simulink model "gm_filter_low_pass_simulink"  (R2025a)
settings: Solver=FixedStepAuto  StartTime=0.0  StopTime=10e-3  MaxStep=1/(44e3)  RelTol=1e-3  EnableMultiTasking=on
settings Model: Creator=thiag  LastModifiedBy=thiag
settings SolverCC: PositivePriorityOrder=on
settings OptimizationCC: BlockReduction=off  ConditionallyExecuteInputs=off  DefaultParameterBehavior=Inlined  UseDivisionForNetSlopeComputation=on  GainParamInheritBuiltInType=on  DefaultUnderspecifiedDataType=single  EnhancedBackFolding=on  PassReuseOutputArgsAs=Individual arguments  ZeroExternalMemoryAtStartup=off  ZeroInternalMemoryAtStartup=off  MaxStackSize=64  OptimizeBlockOrder=speed  DifferentSizesBufferReuse=on  OptimizationCustomize=off  EfficientTunableParamExpr=on
settings DebuggingCC: InheritedTsInSrcMsg=none  ParameterTunabilityLossMsg=error
settings HardwareCC: ProdBitPerPointer=32.0  ProdBitPerSizeT=32.0  ProdBitPerPtrDiffT=32.0  ProdLargestAtomicInteger=Long  ProdLargestAtomicFloat=Double  ProdWordSize=32.0  ProdLongLongMode=on  ProdHWDeviceType=ARM Compatible->ARM Cortex-A (32-bit)
settings SFSimCC: MATLABDynamicMemAlloc=off
settings RTWCC: SystemTargetFile=ert.tlc  HardwareBoard=Arrow SoCKit development board  TLCOptions="-aInlineSetEventsForThisBaseRateFcn=TLC_FALSE -aSuppressMultiTaskScheduler=TLC_FALSE  -aRateBasedStepFcn=0"  TemplateMakefile=ert_default_tmf  GenerateReport=on  Toolchain=ARM Development Studio Altera Edition (DS-5 AE)  LaunchReport=on  GenerateWebview=on  Description=Embedded Coder
settings CodeAppCC: ForceParamTrailComments=on  IgnoreCustomStorageClasses=off  OperatorAnnotations=on  SimulinkDataObjDesc=on  SFDataObjDesc=on  InsertBlockDesc=on
settings ERTTargetCC: ExtModeTransport=0.0  ExtModeStaticAlloc=off  ExtModeMexFile=ext_comm  ExtModeIntrfLevel=Level1

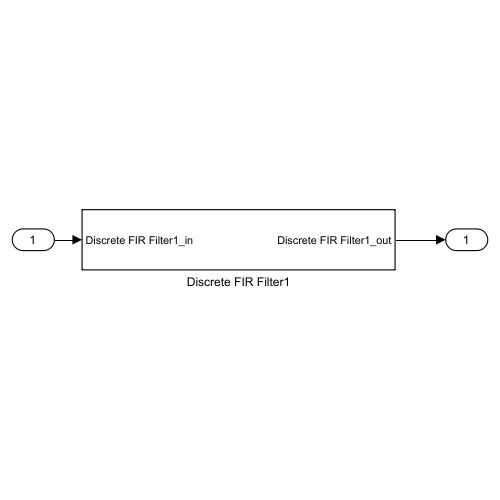
[thumbnail: Simulink's stored preview of the top-level diagram]
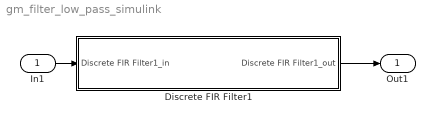
== system gm_filter_low_pass_simulink ==
  In1 : Inport  OutDataTypeStr=single  PortDimensions=1  SampleTime=0.0002
  Discrete FIR Filter1 : Subsystem
  Out1 : Outport  SampleTime=0.0002  VectorParamsAs1DForOutWhenUnconnected=off
  wires:
  In1/1 -> Discrete FIR Filter1/1(Discrete FIR Filter1_in)
  Discrete FIR Filter1/1(Discrete FIR Filter1_out) -> Out1/1

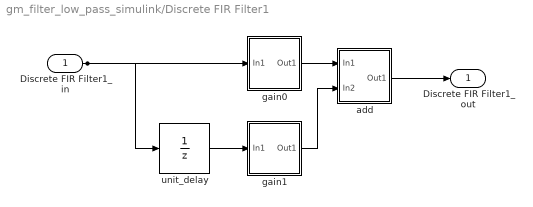
== system gm_filter_low_pass_simulink/Discrete FIR Filter1 ==
  Discrete FIR Filter1_in : Inport  OutDataTypeStr=single  SampleTime=0.0002
  add : Subsystem
      mask Display: disp('NFP\nadd');
  gain0 : Subsystem
      mask Display: disp('NFP\ngain_pow2');
  gain1 : Subsystem
      mask Display: disp('NFP\ngain_pow2');
  unit_delay : UnitDelay  InitialCondition=double(0)  SampleTime=0.0002
  Discrete FIR Filter1_out : Outport  OutDataTypeStr=single  SampleTime=0.0002
  wires:
  Discrete FIR Filter1_in/1 -> gain0/1(In1), unit_delay/1
  unit_delay/1 -> gain1/1(In1)
  gain0/1(Out1) -> add/1(In1)
  add/1(Out1) -> Discrete FIR Filter1_out/1
  gain1/1(Out1) -> add/2(In2)

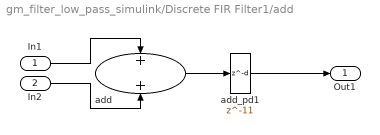
== system gm_filter_low_pass_simulink/Discrete FIR Filter1/add ==
  In1 : Inport
  In2 : Inport  Port=2
  add : Sum  OutDataTypeStr=single  SampleTime=0.0002
  add_pd1 : Delay  DelayLength=11
  Out1 : Outport
  wires:
  In1/1 -> add/1
  In2/1 -> add/2
  add/1 -> add_pd1/1
  add_pd1/1 -> Out1/1

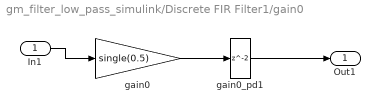
== system gm_filter_low_pass_simulink/Discrete FIR Filter1/gain0 ==
  In1 : Inport
  gain0 : Gain  Gain=single(0.5)
  gain0_pd1 : Delay
  Out1 : Outport
  wires:
  In1/1 -> gain0/1
  gain0/1 -> gain0_pd1/1
  gain0_pd1/1 -> Out1/1

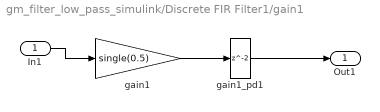
== system gm_filter_low_pass_simulink/Discrete FIR Filter1/gain1 ==
  In1 : Inport
  gain1 : Gain  Gain=single(0.5)
  gain1_pd1 : Delay
  Out1 : Outport
  wires:
  In1/1 -> gain1/1
  gain1/1 -> gain1_pd1/1
  gain1_pd1/1 -> Out1/1
